simulink model "Modelka_2"  (Simulink 4.00)
settings: Solver=ode45  StartTime=0.0  StopTime=10.0  RelTol=1e-3
settings Model: LastModifiedBy=user

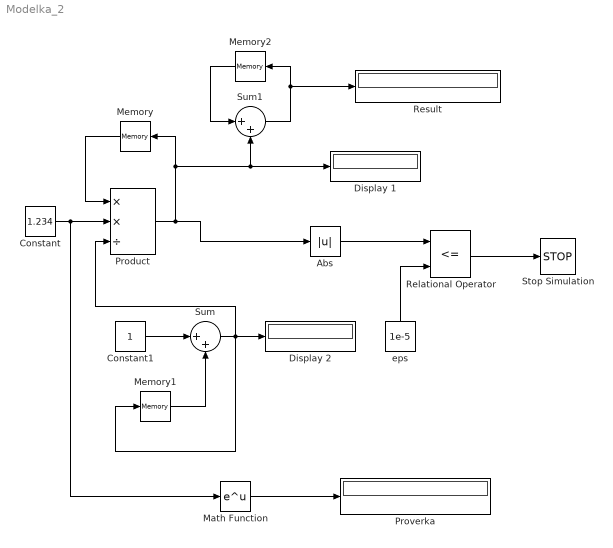
== system Modelka_2 ==
  Abs : Abs  SaturateOnIntegerOverflow=on
  Constant : Constant  Value=1.234
  Constant1 : Constant  Value=1
  Display 1 : Display
      settings: Format=short
  Display 2 : Display
      settings: Format=short
  Math Function : Math  Operator=exp  OutputSignalType=auto
  Memory : Memory  Orientation=left  X0=1  InheritSampleTime=off
      settings: RTWStateStorageClass=Auto
  Memory1 : Memory  X0=0  InheritSampleTime=off
      settings: RTWStateStorageClass=Auto
  Memory2 : Memory  Orientation=left  X0=1  InheritSampleTime=off
      settings: RTWStateStorageClass=Auto
  Product : Product  Inputs=**/  Multiplication=Element-wise(.*)  SaturateOnIntegerOverflow=on
  Proverka : Display
  Relational Operator : RelationalOperator  Operator=<=
  Result : Display
  Stop Simulation : Stop
  Sum : Sum  Inputs=|++  SaturateOnIntegerOverflow=on
  Sum1 : Sum  Inputs=|++  SaturateOnIntegerOverflow=on
  eps : Constant  Orientation=up  Value=1e-5
  wires:
  Constant/1 -> Product/2, Math Function/1
  Memory/1 -> Product/1
  Constant1/1 -> Sum/1
  Memory1/1 -> Sum/2
  Sum/1 -> Display 2/1, Memory1/1, Product/3
  Product/1 -> Abs/1, Memory/1, Display 1/1, Sum1/2
  Sum1/1 -> Memory2/1, Result/1
  Memory2/1 -> Sum1/1
  Abs/1 -> Relational Operator/1
  eps/1 -> Relational Operator/2
  Math Function/1 -> Proverka/1
  Relational Operator/1 -> Stop Simulation/1
